simulink model "lecture_longitudinal_model_model"  (R2016b)
settings: Solver=ode45  StartTime=0.0  StopTime=60  RelTol=1e-3  EnableMultiTasking=on
values from neighbouring files (symbols this model uses):
  Along = temp.Along    [lecture_longitudinal_model.m]    (also in longitudinal_linear_model.mat = [-0.035373280601 -0.220315996557 -0.00101370763635 0 0.06117)
  Blong = temp.Blong    [lecture_longitudinal_model.m]    (also in longitudinal_linear_model.mat = [0 0 0 0 0.109430402517 -7.31573284914 -2.91927108265 0 0 0 )
  Clong = eye(4)    [lecture_longitudinal_model.m]
  DeltaXlong0 = [0;0;0;3*pi/180]    [lecture_longitudinal_model.m]
  Dlong = zeros(4,5)    [lecture_longitudinal_model.m]
  doublet_duration = 1    [lecture_longitudinal_model.m]
  doublet_magnitude = 2*pi/180    (= 0.0349065850399)    [lecture_longitudinal_model.m]
  doublet_time = 15    [lecture_longitudinal_model.m]
settings Model: Creator=lum  LastModifiedBy=chris
settings DataIOCC: LimitDataPoints=on  SaveFormat=Array  SignalLoggingSaveFormat=ModelDataLogs
settings OptimizationCC: ExpressionDepthLimit=2147483647  InitFltsAndDblsToZero=on  LifeSpan=inf
settings DebuggingCC: SaveWithParameterizedLinksMsg=none  UnderspecifiedInitializationDetection=Classic  MergeDetectMultiDrivingBlocksExec=none  SignalResolutionControl=TryResolveAllWithWarning  SolverPrmCheckMsg=warning  MultiTaskDSMMsg=warning  MultiTaskCondExecSysMsg=none  FcnCallInpInsideContextMsg=warning  StateNameClashWarn=warning  SFUnexpectedBacktrackingDiag=warning  SFNoUnconditionalDefaultTransitionDiag=warning  SFExecutionAtInitializationDiag=none
settings HardwareCC: ProdBitPerPointer=32  ProdBitPerSizeT=32  ProdBitPerPtrDiffT=32  ProdLargestAtomicFloat=None  ProdIntDivRoundTo=Undefined  ProdEndianess=Unspecified  ProdWordSize=32  ProdHWDeviceType=32-bit Generic
settings ModelReferenceCC: PropagateSignalLabelsOutOfModel=off
settings GRTTargetCC: TargetFcnLib=ansi_tfl_tmw.mat  TargetLangStandard=C89/C90 (ANSI)  GeneratePreprocessorConditionals=Disable all  CombineOutputUpdateFcns=off  GRTInterface=on
settings ConfigComp: CovMetricSettings=dw  CovHtmlReporting=on  CovSaveCumulativeToWorkspaceVar=on  CovSaveSingleToWorkspaceVar=on  CovExternalEMLEnable=off

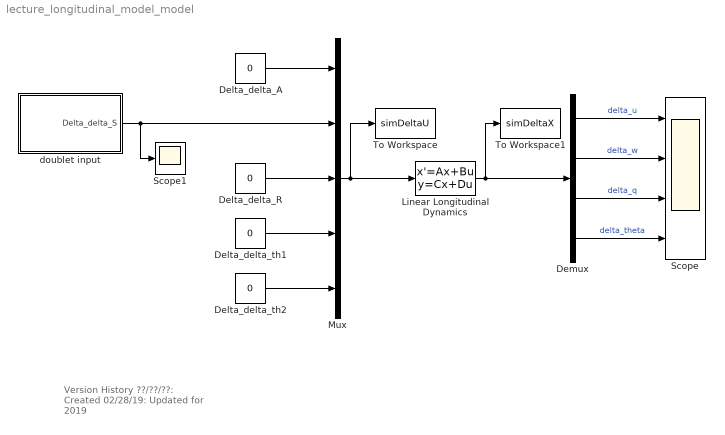
== system lecture_longitudinal_model_model ==
  note: Version History
      | ??/??/??: Created
      | 02/28/19: Updated for 2019
  Delta_delta_A : Constant  Value=0
  Delta_delta_R : Constant  Value=0
  Delta_delta_th1 : Constant  Value=0
  Delta_delta_th2 : Constant  Value=0
  Demux : Demux
  Linear Longitudinal Dynamics : StateSpace  A=Along  B=Blong  C=Clong  D=Dlong  X0=DeltaXlong0
  Mux : Mux  Inputs=5
  Scope : Scope  NumInputPorts=4
  Scope1 : Scope
  To Workspace : ToWorkspace  VariableName=simDeltaU  SaveFormat=Structure With Time  SampleTime=-1
  To Workspace1 : ToWorkspace  VariableName=simDeltaX  SaveFormat=Structure With Time  SampleTime=-1
  doublet input : Subsystem
  wires:
  Mux/1 -> Linear Longitudinal Dynamics/1, To Workspace/1
  Linear Longitudinal Dynamics/1 -> Demux/1, To Workspace1/1
  Delta_delta_A/1 -> Mux/1
  Delta_delta_R/1 -> Mux/3
  Delta_delta_th1/1 -> Mux/4
  Delta_delta_th2/1 -> Mux/5
  Demux/1 -> Scope/1  "delta_u"
  Demux/2 -> Scope/2  "delta_w"
  Demux/3 -> Scope/3  "delta_q"
  Demux/4 -> Scope/4  "delta_theta"
  doublet input/1(Delta_delta_S) -> Mux/2, Scope1/1

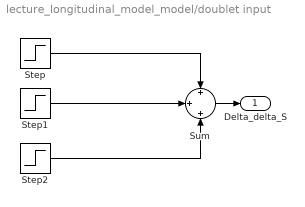
== system lecture_longitudinal_model_model/doublet input ==
  Step : Step  Time=doublet_time  After=doublet_magnitude  SampleTime=0
  Step1 : Step  Time=doublet_time+doublet_duration  After=-2*doublet_magnitude  SampleTime=0
  Step2 : Step  Time=doublet_time+2*doublet_duration  After=doublet_magnitude  SampleTime=0
  Sum : Sum  Inputs=+|+|+
  Delta_delta_S : Outport
  wires:
  Step/1 -> Sum/1
  Step1/1 -> Sum/2
  Step2/1 -> Sum/3
  Sum/1 -> Delta_delta_S/1
